simulink model "j2s"  (R2023b)
settings: Solver=VariableStepAuto  StartTime=0.0  StopTime=10.0  RelTol=1e-3
settings Model: Creator=asus  LastModifiedBy=asus

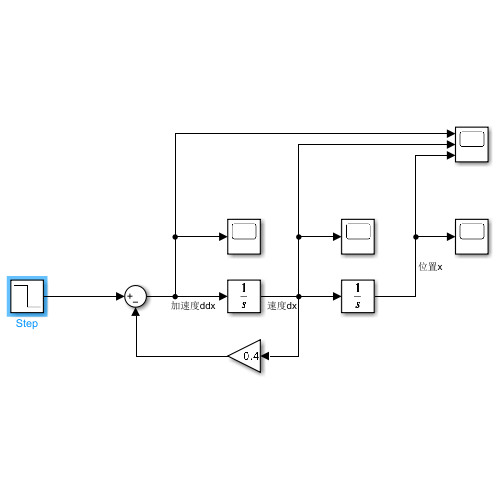
[thumbnail: Simulink's stored preview of the top-level diagram]
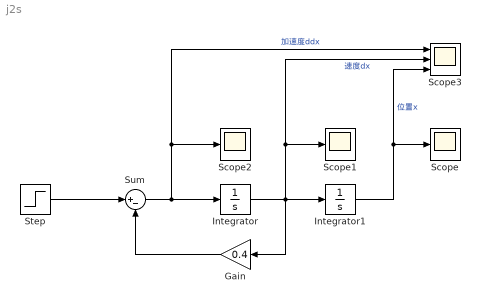
== system j2s ==
  Gain : Gain  Gain=0.4
  Integrator : Integrator
  Integrator1 : Integrator
  Scope : Scope
  Scope1 : Scope
  Scope2 : Scope
  Scope3 : Scope  NumInputPorts=3
  Step : Step  Time=2  Before=1  After=0  SampleTime=0
  Sum : Sum  Inputs=|+-
  wires:
  Integrator/1 -> Scope3/2, Scope1/1, Gain/1, Integrator1/1  "速度dx"
  Integrator1/1 -> Scope3/3, Scope/1  "位置x"
  Sum/1 -> Scope3/1, Scope2/1, Integrator/1  "加速度ddx"
  Step/1 -> Sum/1
  Gain/1 -> Sum/2
